simulink model "problem5circuit"  (R2020b)
settings: Solver=VariableStepAuto  StartTime=0.0  StopTime=10.0  RelTol=1e-3
settings Model: Creator=Shivashis  LastModifiedBy=Shivashis

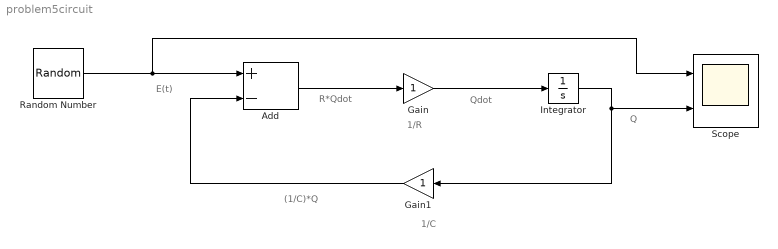
== system problem5circuit ==
  note: (1/C)*Q
  note: R*Qdot
  note: 1/C
  note: E(t)
  note: Q
  note: 1/R
  note: Qdot
  Add : Sum  Inputs=+-
  Gain : Gain
  Gain1 : Gain
  Integrator : Integrator
  Random Number : RandomNumber  SampleTime=0.1
  Scope : Scope  NumInputPorts=2
  wires:
  Integrator/1 -> Scope/2, Gain1/1
  Gain1/1 -> Add/2
  Add/1 -> Gain/1
  Random Number/1 -> Scope/1, Add/1
  Gain/1 -> Integrator/1
